simulink library "turbine_ul"  (R2018b)
settings: Solver=VariableStepAuto  StartTime=0.0  StopTime=10.0  RelTol=1e-3
libraries: vrlib x2
settings Model: Creator=mcobb  LastModifiedBy=mcobb

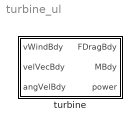
== system turbine_ul ==
  turbine : Subsystem  mask{diam=0, Cp=0, Cd=0, rho=0, rTurb=[0 1 0]}
      mask prompts: diam "Diameter"; Cp "Power Coefficient"; Cd "Drag Coefficient"; rho "Density"; rTurb "Turbine position vec"

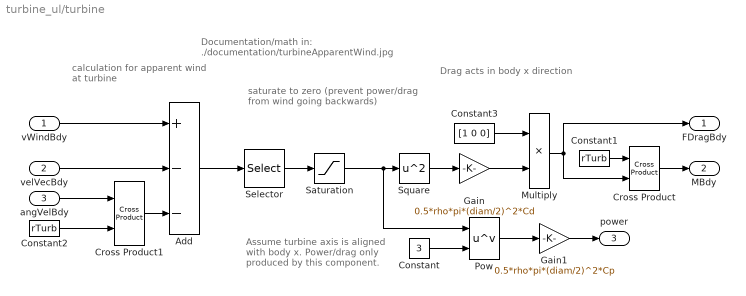
== system turbine_ul/turbine ==
  note: Documentation/math in:
      | ./documentation/turbineApparentWind.jpg
  note: calculation for
      | apparent wind at turbine
  note: Drag acts in
      | body x direction
  note: saturate to zero (prevent power/drag
      | from wind going backwards)
  note: Assume turbine axis
      | is aligned with body x.
      | Power/drag only produced
      | by this component.
  vWindBdy : Inport
  velVecBdy : Inport  Port=2
  angVelBdy : Inport  Port=3
  Add : Sum  Inputs=+--
  Constant : Constant  Value=3
  Constant1 : Constant  Value=rTurb
  Constant2 : Constant  Value=rTurb
  Constant3 : Constant  Value=[1 0 0]
  Cross Product : vrlib/Utilities/Cross Product
      settings: SourceProductBaseCode=VR
  Cross Product1 : vrlib/Utilities/Cross Product
      settings: SourceProductBaseCode=VR
  Gain : Gain  Gain=0.5*rho*pi*(diam/2)^2*Cd
  Gain1 : Gain  Gain=0.5*rho*pi*(diam/2)^2*Cp
  Multiply : Product
  Pow : Math  Operator=pow  RndMeth=Zero  SaturateOnIntegerOverflow=on
  Saturation : Saturate  UpperLimit=inf  LowerLimit=0
  Selector : Selector  InputPortWidth=3  IndexOptions=Index vector (dialog)  Indices=1  OutputSizes=1
  Square : Math  Operator=square  SaturateOnIntegerOverflow=on
  FDragBdy : Outport
  MBdy : Outport  Port=2
  power : Outport  Port=3
  wires:
  Selector/1 -> Saturation/1
  Square/1 -> Gain/1
  Gain/1 -> Multiply/2
  Multiply/1 -> FDragBdy/1, Cross Product/2
  Gain1/1 -> power/1
  Saturation/1 -> Pow/1, Square/1
  Constant1/1 -> Cross Product/1
  Cross Product/1 -> MBdy/1
  vWindBdy/1 -> Add/1
  angVelBdy/1 -> Cross Product1/1
  Constant2/1 -> Cross Product1/2
  Add/1 -> Selector/1
  Constant3/1 -> Multiply/1
  velVecBdy/1 -> Add/2
  Cross Product1/1 -> Add/3
  Pow/1 -> Gain1/1
  Constant/1 -> Pow/2
